simulink model "PIDcranesimu"  (R2015a)
settings: Solver=ode45  StartTime=0.0  StopTime=30  RelTol=1e-3
values from neighbouring files (symbols this model uses):
  k = 5    [alternateDesign.m]    (also in controllerDesign.m = 10; ekstraLoop.m = 3.46; ekstranul.m = 2)
undefined symbols (not defined in the file or in its folder): Td, Ti, Tp
libraries: cstblocks x7, simulink x1
settings Model: Creator=Steffan  LastModifiedBy=Steffan

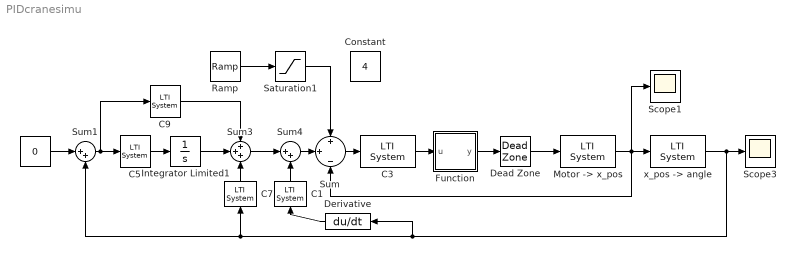
== system PIDcranesimu ==
  " " : Constant  Value=0
  C1 : cstblocks/LTI System  sys=Td*k  IC=[]
  C3 : cstblocks/LTI System  sys=C2  IC=[]
  C5 : cstblocks/LTI System  sys=k/Ti  IC=[]
  C7 : cstblocks/LTI System  sys=k  IC=[]
  C9 : cstblocks/LTI System  sys=Tp*k  IC=[]
  Constant : Constant  Value=4
  Dead Zone : DeadZone  LowerValue=-4.5  UpperValue=4.5  SaturateOnIntegerOverflow=on
  Derivative : Derivative
  Function : MATLAB Function  TreatAsAtomicUnit=on
  Integrator Limited1 : Integrator  LimitOutput=on  UpperSaturationLimit=1  LowerSaturationLimit=-1
  "Motor -> x_pos" : cstblocks/LTI System  sys=X  IC=[]
  Ramp : simulink/Sources/Ramp  slope=.5  start=0  X0=0
  Saturation1 : Saturate  UpperLimit=4  LowerLimit=0
  Scope1 : Scope
  Scope3 : Scope
      settings: SaveName=ScopeData2
  Sum : Sum  Inputs=+|+|-
  Sum1 : Sum  Inputs=|++
  Sum3 : Sum  Inputs=+++
  Sum4 : Sum  Inputs=|++
  "x_pos -> angle" : cstblocks/LTI System  sys=W  IC=[]
  wires:
  " "/1 -> Sum1/1
  "x_pos -> angle"/1 -> Scope3/1, Derivative/1, Sum1/2, C7/1
  Integrator Limited1/1 -> Sum3/2
  Sum4/1 -> Sum/2
  Sum3/1 -> Sum4/1
  C1/1 -> Sum4/2
  Derivative/1 -> C1/1
  Sum1/1 -> C5/1, C9/1
  Ramp/1 -> Saturation1/1
  Saturation1/1 -> Sum/1
  Function/1(y) -> Dead Zone/1
  C9/1 -> Sum3/1
  Sum/1 -> C3/1
  C5/1 -> Integrator Limited1/1
  "Motor -> x_pos"/1 -> Scope1/1, Sum/3, "x_pos -> angle"/1
  C3/1 -> Function/1(u)
  C7/1 -> Sum3/3
  Dead Zone/1 -> "Motor -> x_pos"/1

== matlab function PIDcranesimu/Function ==
  data: u input; y output
function y = fcn(u)
if (u > -4.6 && u < -0.2)
        u = -4.6;
elseif (u < 4.6 && u > 0.2)
        u = 4.6;
elseif (u > 12.5) 
        u = 12.5;
elseif (u < -12.5) 
        u = -12.5;
    end;    
y = u;
